simulink model "limbControlPID"  (R2018b)
settings: Solver=FixedStepAuto  StartTime=0.0  StopTime=300  FixedStep=Ts  RelTol=1e-3
InitFcn:
  | init
undefined symbols (not defined in the file or in its folder): B1, B2, B3, g, J, K1, K2, K3, l, m, PID_MPT, Td
libraries: simulink x3
settings Model: Creator=hhhhh  LastModifiedBy=root

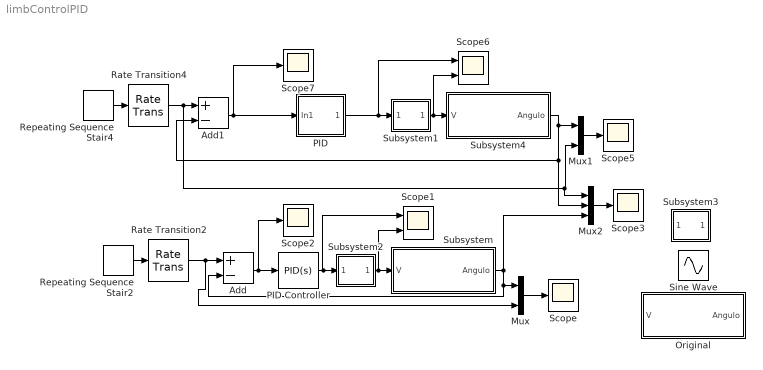
== system limbControlPID ==
  Add : Sum  Inputs=+-
  Add1 : Sum  Inputs=+-
  Mux : Mux  Inputs=2
  Mux1 : Mux  Inputs=2
  Mux2 : Mux  Inputs=3
  Original : Subsystem
  PID : Subsystem
  PID Controller : simulink/Continuous/PID Controller  Controller=PID  Form=Ideal  TimeDomain=Continuous-time  SampleTime=-1  IntegratorMethod=Forward Euler  FilterMethod=Forward Euler  ControllerParametersSource=internal  P=4.590499090756  I=1.042343403683  D=0.375822570602048  UseFilter=on  N=200  TunerSelectOption=Transfer Function Based (PID Tuner App)  InitialConditionSource=internal  InitialConditionForIntegrator=0  InitialConditionForFilter=0  DifferentiatorICPrevScaledInput=0  ExternalReset=none  TrackingMode=off  Kt=1  LimitOutput=on  UpperSaturationLimit=1.35  LowerSaturationLimit=0  LinearizeAsGain=on  AntiWindupMode=none  Kb=1  POutMin=[]  POutMax=[]  IOutMin=[]  IOutMax=[]  DOutMin=[]  DOutMax=[]  NOutMin=[]  NOutMax=[]  SumOutMin=[]  SumOutMax=[]  SaturationOutMin=[]  SaturationOutMax=[]  PParamMin=[]  PParamMax=[]  IParamMin=[]  IParamMax=[]  DParamMin=[]  DParamMax=[]  NParamMin=[]  NParamMax=[]  KbParamMin=[]  KbParamMax=[]  KtParamMin=[]  KtParamMax=[]  KbOutMin=[]  KbOutMax=[]  KtOutMin=[]  KtOutMax=[]  IntegratorOutMin=[]  IntegratorOutMax=[]  FilterOutMin=[]  FilterOutMax=[]  SumI1OutMin=[]  SumI1OutMax=[]  SumI2OutMin=[]  SumI2OutMax=[]  SumI3OutMin=[]  SumI3OutMax=[]  SumI4OutMin=[]  SumI4OutMax=[]  SumDOutMin=[]  SumDOutMax=[]  DifferentiatorOutMin=[]  DifferentiatorOutMax=[]  FilterDiffOutCoefMin=[]  FilterDiffOutCoefMax=[]  ReciprocalOutMin=[]  ReciprocalOutMax=[]  SumDenOutMin=[]  SumDenOutMax=[]  SumNumOutMin=[]  SumNumOutMax=[]  DivideOutMin=[]  DivideOutMax=[]  IntegratorContinuousStateAttributes=''  IntegratorStateMustResolveToSignalObject=off  IntegratorRTWStateStorageClass=Auto  FilterContinuousStateAttributes=''  FilterStateMustResolveToSignalObject=off  FilterRTWStateStorageClass=Auto  ParallelPVariant=Passthrough  IdealPVariant=InternalParameters  IVariant=InternalParameters  DVariant=InternalParameters  IntegratorVariant=Continuous  SatVariant=Enabled  AWVariant=Passthrough  PCopyVariant=Disabled  TRVariant=Disabled  FdbkBlocksVariant=Forward  IdealPFdbkVariant=Disabled  SatFdbkVariant=Disabled  DerivativeFilterVariant=ContFilter  NVariant=InternalParameters  NCopyVariant=Disabled  FilterICVariant=InternalICsFilter  IntegratorICVariant=InternalICs  ExternalResetVariant=Disabled  TRSumVariant=Passthrough  SumFdbkVariant=Disabled  SumVariant=Sum_PID
  Rate Transition2 : RateTransition
  Rate Transition4 : RateTransition
  Repeating Sequence Stair2 : simulink/Sources/Repeating Sequence Stair  OutValues="1.3*[0\t0.0523359562429438\t0.104528463267653\t0.156434465040231\t0.207911690817759\t0.258819045102521\t0.309016994374947\t0.358367949545300\t0.406736643075800\t0.453990499739547\t0.500000000000000\t0.544639035015027\t0.587785252292473\t0.629320391049837\t0.669130606358858\t0.707106781186548\t0.743144825477394\t0.777145961456971\t0.809016994374948\t0.838670567945424\t0.866025403784439\t0.891006524188368\t0.913545457642601\t0.933580426497202\t0.951056516295154\t0.965925826289068\t0.978147600733806\t0.987688340595138\t0.994521895368273\t0.998629534754574\t1\t0.998629534754574\t0.994521895368273\t0.987688340595138\t0.978147600733806\t0.965925826289068\t0.951056516295154\t0.933580426497202\t0.913545457642601\t0.891006524188368\t0.866025403784439\t0.838670567945424\t0.809016994374948\t0.777145961456971\t0.743144825477394\t0.707106781186548\t0.669130606358858\t0.629320391049837\t0.587785252292473\t0.544639035015027\t0.500000000000000\t0.453990499739547\t0.406736643075800\t0.358367949545300\t0.309016994374948\t0.258819045102521\t0.207911690817759\t0.156434465040231\t0.104528463267654\t0.0523359562429438].'"  tsamp=4  OutMin=[]  OutMax=[]  OutDataTypeStr=double  OutputDataTypeScalingMode=double  OutDataType=fixdt(0,8)  ConRadixGroup=Best Precision: Vector-wise  OutScaling=2^-12
  Repeating Sequence Stair4 : simulink/Sources/Repeating Sequence Stair  OutValues="1.3*[0\t0.0523359562429438\t0.104528463267653\t0.156434465040231\t0.207911690817759\t0.258819045102521\t0.309016994374947\t0.358367949545300\t0.406736643075800\t0.453990499739547\t0.500000000000000\t0.544639035015027\t0.587785252292473\t0.629320391049837\t0.669130606358858\t0.707106781186548\t0.743144825477394\t0.777145961456971\t0.809016994374948\t0.838670567945424\t0.866025403784439\t0.891006524188368\t0.913545457642601\t0.933580426497202\t0.951056516295154\t0.965925826289068\t0.978147600733806\t0.987688340595138\t0.994521895368273\t0.998629534754574\t1\t0.998629534754574\t0.994521895368273\t0.987688340595138\t0.978147600733806\t0.965925826289068\t0.951056516295154\t0.933580426497202\t0.913545457642601\t0.891006524188368\t0.866025403784439\t0.838670567945424\t0.809016994374948\t0.777145961456971\t0.743144825477394\t0.707106781186548\t0.669130606358858\t0.629320391049837\t0.587785252292473\t0.544639035015027\t0.500000000000000\t0.453990499739547\t0.406736643075800\t0.358367949545300\t0.309016994374948\t0.258819045102521\t0.207911690817759\t0.156434465040231\t0.104528463267654\t0.0523359562429438].'"  tsamp=4  OutMin=[]  OutMax=[]  OutDataTypeStr=double  OutputDataTypeScalingMode=double  OutDataType=fixdt(0,8)  ConRadixGroup=Best Precision: Vector-wise  OutScaling=2^-12
  Scope{,2..3,5,7} (5 alike) : Scope
  Scope1 : Scope  NumInputPorts=2
  Scope6 : Scope  NumInputPorts=2
  Sine Wave : Sin  SampleTime=0
  Subsystem : Subsystem
  Subsystem1 : Subsystem
  Subsystem2 : Subsystem
  Subsystem3 : Subsystem
  Subsystem4 : Subsystem
  wires:
  Rate Transition2/1 -> Add/1, Mux/2
  Subsystem/1(Angulo) -> Mux2/3, Mux/1, Add/2
  Add/1 -> Scope2/1, PID Controller/1
  Mux/1 -> Scope/1
  PID Controller/1 -> Scope1/1, Subsystem2/1(In1)
  Subsystem2/1(Out1) -> Scope1/2, Subsystem/1(V)
  Repeating Sequence Stair2/1 -> Rate Transition2/1
  Subsystem1/1(Out1) -> Subsystem4/1(V), Scope6/2
  Mux1/1 -> Scope5/1
  Repeating Sequence Stair4/1 -> Rate Transition4/1
  Subsystem4/1(Angulo) -> Mux1/1, Mux2/2, Add1/2
  Rate Transition4/1 -> Mux2/1, Mux1/2, Add1/1
  PID/1(Out1) -> Scope6/1, Subsystem1/1(In1)
  Add1/1 -> PID/1(In1), Scope7/1
  Mux2/1 -> Scope3/1

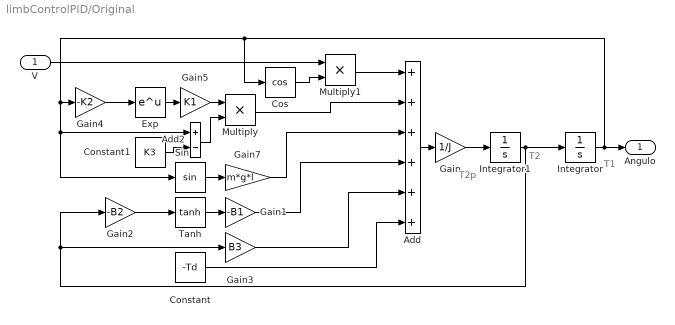
== system limbControlPID/Original ==
  note: T1
  note: T2p
  note: T2
  V : Inport
  Add : Sum  Inputs=++++++
  Add2 : Sum  Inputs=+-
  Constant : Constant  Value=-Td
  Constant1 : Constant  Value=K3
  Cos : Trigonometry  Operator=cos
  Exp : Math  SaturateOnIntegerOverflow=on
  Gain : Gain  Gain=1/J
  Gain1 : Gain  Gain=-B1
  Gain2 : Gain  Gain=-B2
  Gain3 : Gain  Gain=B3
  Gain4 : Gain  Gain=-K2
  Gain5 : Gain  Gain=K1
  Gain7 : Gain  Gain=m*g*l
  Integrator : Integrator
  Integrator1 : Integrator
  Multiply : Product
  Multiply1 : Product
  Sin : Trigonometry
  Tanh : Trigonometry  Operator=tanh
  Angulo : Outport
  wires:
  Integrator/1 -> Gain4/1, Add2/1, Sin/1, Cos/1, Angulo/1
  Gain2/1 -> Tanh/1
  Integrator1/1 -> Gain2/1, Gain3/1, Integrator/1
  Exp/1 -> Gain5/1
  Gain7/1 -> Add/3
  Sin/1 -> Gain7/1
  V/1 -> Multiply1/1
  Add2/1 -> Multiply/2
  Multiply1/1 -> Add/1
  Gain4/1 -> Exp/1
  Multiply/1 -> Add/2
  Tanh/1 -> Gain1/1
  Add/1 -> Gain/1
  Cos/1 -> Multiply1/2
  Gain3/1 -> Add/5
  Constant/1 -> Add/6
  Gain1/1 -> Add/4
  Gain5/1 -> Multiply/1
  Gain/1 -> Integrator1/1
  Constant1/1 -> Add2/2

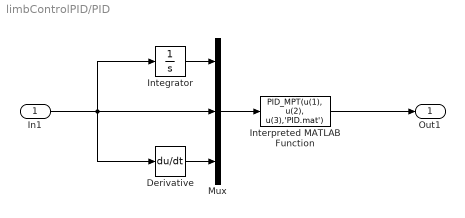
== system limbControlPID/PID ==
  In1 : Inport
  Derivative : Derivative
  Integrator : Integrator
  Interpreted MATLAB Function : MATLABFcn  MATLABFcn=PID_MPT(u(1), u(2), u(3),'PID.mat')  OutputDimensions=1
  Mux : Mux  Inputs=3
  Out1 : Outport
  wires:
  Interpreted MATLAB Function/1 -> Out1/1
  In1/1 -> Integrator/1, Mux/2, Derivative/1
  Mux/1 -> Interpreted MATLAB Function/1
  Integrator/1 -> Mux/1
  Derivative/1 -> Mux/3

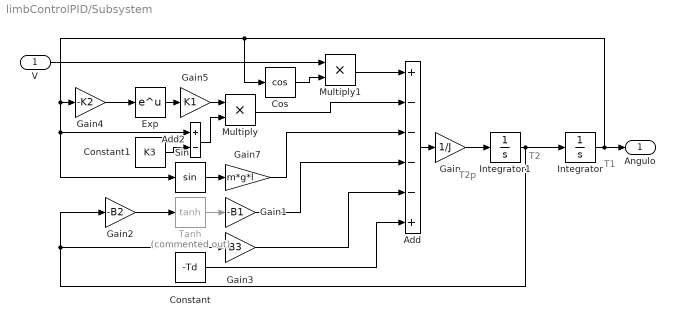
== system limbControlPID/Subsystem ==
  note: T2
  note: T2p
  note: T1
  V : Inport
  Add : Sum  Inputs=+----+
  Add2 : Sum  Inputs=+-
  Constant : Constant  Value=-Td
  Constant1 : Constant  Value=K3
  Cos : Trigonometry  Operator=cos
  Exp : Math  SaturateOnIntegerOverflow=on
  Gain : Gain  Gain=1/J
  Gain1 : Gain  Gain=-B1
  Gain2 : Gain  Gain=-B2
  Gain3 : Gain  Gain=B3
  Gain4 : Gain  Gain=-K2
  Gain5 : Gain  Gain=K1
  Gain7 : Gain  Gain=m*g*l
  Integrator : Integrator
  Integrator1 : Integrator
  Multiply : Product
  Multiply1 : Product
  Sin : Trigonometry
  Tanh : Trigonometry  Commented=on  Operator=tanh
  Angulo : Outport
  wires:
  Constant1/1 -> Add2/2
  Gain/1 -> Integrator1/1
  Gain5/1 -> Multiply/1
  Gain1/1 -> Add/4
  Constant/1 -> Add/6
  Gain3/1 -> Add/5
  Cos/1 -> Multiply1/2
  Add/1 -> Gain/1
  Tanh/1 -> Gain1/1
  Multiply/1 -> Add/2
  Gain4/1 -> Exp/1
  Multiply1/1 -> Add/1
  Add2/1 -> Multiply/2
  V/1 -> Multiply1/1
  Sin/1 -> Gain7/1
  Gain7/1 -> Add/3
  Exp/1 -> Gain5/1
  Integrator1/1 -> Integrator/1, Gain3/1, Gain2/1
  Gain2/1 -> Tanh/1
  Integrator/1 -> Angulo/1, Cos/1, Sin/1, Add2/1, Gain4/1

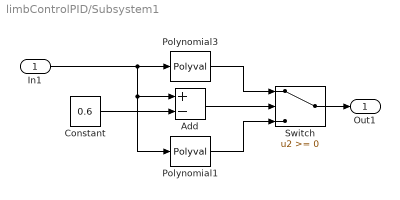
== system limbControlPID/Subsystem1 ==
  In1 : Inport
  Add : Sum  Inputs=+-
  Constant : Constant  Value=0.6
  Polynomial1 : Polyval  Coefs=|
      | [0
      | 0
      | 0
      | 4.96473696106646
      | 0
      | 1.22506777764656
      | 11.8762695363768
      | 0]
  Polynomial3 : Polyval  Coefs=|
      | [1334.93659745298
      | -7873.77408130260
      | 19679.6581173489
      | -26904.1335294621
      | 21674.5719980287
      | -10255.6450049827
      | 2645.19572957251
      | -282.136494548769]
  Switch : Switch
  Out1 : Outport
  wires:
  Switch/1 -> Out1/1
  In1/1 -> Add/1, Polynomial1/1, Polynomial3/1
  Constant/1 -> Add/2
  Add/1 -> Switch/2
  Polynomial3/1 -> Switch/1
  Polynomial1/1 -> Switch/3

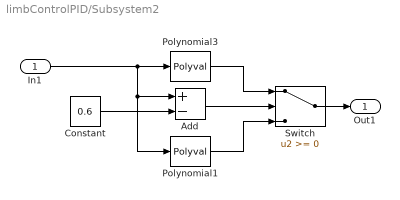
== system limbControlPID/Subsystem2 ==
  In1 : Inport
  Add : Sum  Inputs=+-
  Constant : Constant  Value=0.6
  Polynomial1 : Polyval  Coefs=|
      | [0
      | 0
      | 0
      | 4.96473696106646
      | 0
      | 1.22506777764656
      | 11.8762695363768
      | 0]
  Polynomial3 : Polyval  Coefs=|
      | [1334.93659745298
      | -7873.77408130260
      | 19679.6581173489
      | -26904.1335294621
      | 21674.5719980287
      | -10255.6450049827
      | 2645.19572957251
      | -282.136494548769]
  Switch : Switch
  Out1 : Outport
  wires:
  Polynomial1/1 -> Switch/3
  Polynomial3/1 -> Switch/1
  Add/1 -> Switch/2
  Constant/1 -> Add/2
  In1/1 -> Polynomial3/1, Polynomial1/1, Add/1
  Switch/1 -> Out1/1

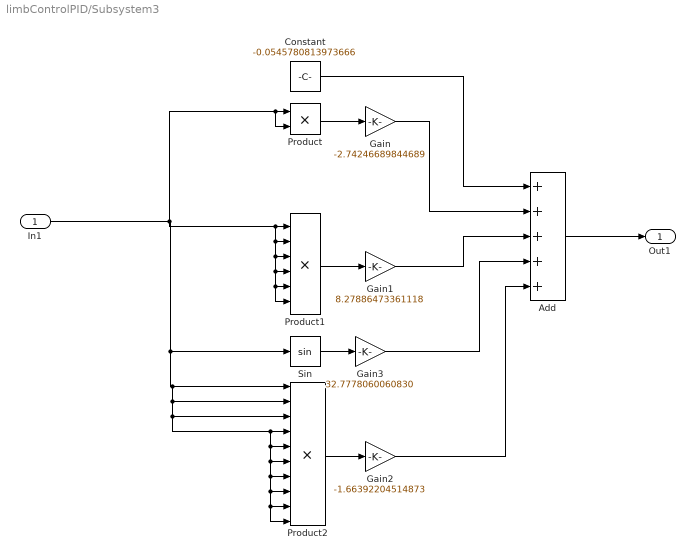
== system limbControlPID/Subsystem3 ==
  In1 : Inport
  Add : Sum  Inputs=+++++
  Constant : Constant  Value=-0.0545780813973666
  Gain : Gain  Gain=-2.74246689844689
  Gain1 : Gain  Gain=8.27886473361118
  Gain2 : Gain  Gain=-1.66392204514873
  Gain3 : Gain  Gain=32.7778060060830
  Product : Product
  Product1 : Product  Inputs=6
  Product2 : Product  Inputs=10
  Sin : Trigonometry
  Out1 : Outport
  wires:
  Add/1 -> Out1/1
  In1/1 -> Product/2, Product/1, Product1/6, Product1/5, Product1/4, Product1/3, Product1/2, Product1/1, Sin/1, Product2/10, Product2/9, Product2/8, Product2/7, Product2/6, Product2/5, Product2/4, Product2/3, Product2/2, Product2/1
  Product/1 -> Gain/1
  Constant/1 -> Add/1
  Gain/1 -> Add/2
  Product1/1 -> Gain1/1
  Gain1/1 -> Add/3
  Product2/1 -> Gain2/1
  Sin/1 -> Gain3/1
  Gain3/1 -> Add/4
  Gain2/1 -> Add/5

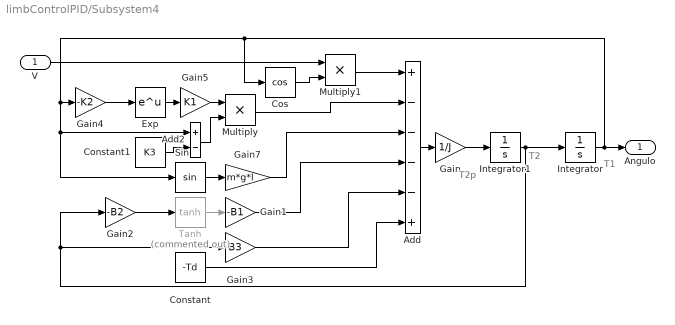
== system limbControlPID/Subsystem4 ==
  note: T1
  note: T2p
  note: T2
  V : Inport
  Add : Sum  Inputs=+----+
  Add2 : Sum  Inputs=+-
  Constant : Constant  Value=-Td
  Constant1 : Constant  Value=K3
  Cos : Trigonometry  Operator=cos
  Exp : Math  SaturateOnIntegerOverflow=on
  Gain : Gain  Gain=1/J
  Gain1 : Gain  Gain=-B1
  Gain2 : Gain  Gain=-B2
  Gain3 : Gain  Gain=B3
  Gain4 : Gain  Gain=-K2
  Gain5 : Gain  Gain=K1
  Gain7 : Gain  Gain=m*g*l
  Integrator : Integrator
  Integrator1 : Integrator
  Multiply : Product
  Multiply1 : Product
  Sin : Trigonometry
  Tanh : Trigonometry  Commented=on  Operator=tanh
  Angulo : Outport
  wires:
  Integrator/1 -> Gain4/1, Add2/1, Sin/1, Cos/1, Angulo/1
  Gain2/1 -> Tanh/1
  Integrator1/1 -> Gain2/1, Gain3/1, Integrator/1
  Exp/1 -> Gain5/1
  Gain7/1 -> Add/3
  Sin/1 -> Gain7/1
  V/1 -> Multiply1/1
  Add2/1 -> Multiply/2
  Multiply1/1 -> Add/1
  Gain4/1 -> Exp/1
  Multiply/1 -> Add/2
  Tanh/1 -> Gain1/1
  Add/1 -> Gain/1
  Cos/1 -> Multiply1/2
  Gain3/1 -> Add/5
  Constant/1 -> Add/6
  Gain1/1 -> Add/4
  Gain5/1 -> Multiply/1
  Gain/1 -> Integrator1/1
  Constant1/1 -> Add2/2
